simulink model "SpeedControl"  (R2023a)
settings: Solver=FixedStepDiscrete  StartTime=0.0  StopTime=inf  FixedStep=0.02  RelTol=1e-3  EnableMultiTasking=on
undefined symbols (not defined in the file or in its folder): DiscIntNeverNeededParam
libraries: arduinolib x3
settings Model: ExtModeTrigDuration=2  Creator=auw_a  LastModifiedBy=auw_a
settings OptimizationCC: EnhancedBackFolding=on  PassReuseOutputArgsAs=Individual arguments  ZeroExternalMemoryAtStartup=off  ZeroInternalMemoryAtStartup=off  MaxStackSize=64  OptimizeBlockOrder=speed  DifferentSizesBufferReuse=on  OptimizationCustomize=off  EfficientTunableParamExpr=on
settings DebuggingCC: ParameterOverflowMsg=none  ParameterTunabilityLossMsg=error
settings HardwareCC: ProdBitPerPointer=32  ProdBitPerSizeT=32  ProdBitPerPtrDiffT=32  ProdLargestAtomicInteger=Long  ProdLargestAtomicFloat=Double  ProdWordSize=32  ProdHWDeviceType=ARM Compatible->ARM Cortex
settings SFSimCC: MATLABDynamicMemAlloc=off
settings RTWCC: Description=Embedded Coder  SystemTargetFile=ert.tlc  HardwareBoard=ESP32-WROOM(Arduino Compatible)  TLCOptions="-aInlineSetEventsForThisBaseRateFcn=TLC_FALSE -aSuppressMultiTaskScheduler=TLC_FALSE  -aRateBasedStepFcn=0"  TemplateMakefile=ert_default_tmf  Toolchain=ESP32  BuildConfiguration=Faster Runs
settings CodeAppCC: ForceParamTrailComments=on  IgnoreCustomStorageClasses=off  OperatorAnnotations=on  SimulinkDataObjDesc=on  SFDataObjDesc=on  InsertBlockDesc=on
settings ERTTargetCC: SupportContinuousTime=on  SupportVariableSizeSignals=on  ExtModeTransport=3  ExtModeStaticAlloc=on  ExtModeAutomaticAllocSize=off  ExtModeStaticAllocSize=65536  ExtModeMexFile=ext_xcp  ExtModeIntrfLevel=Level2 - Open

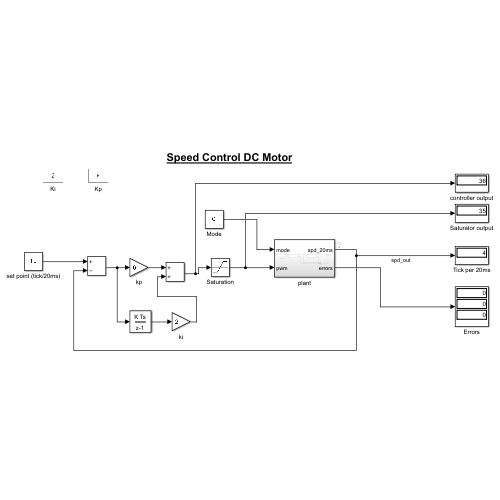
[thumbnail: Simulink's stored preview of the top-level diagram]
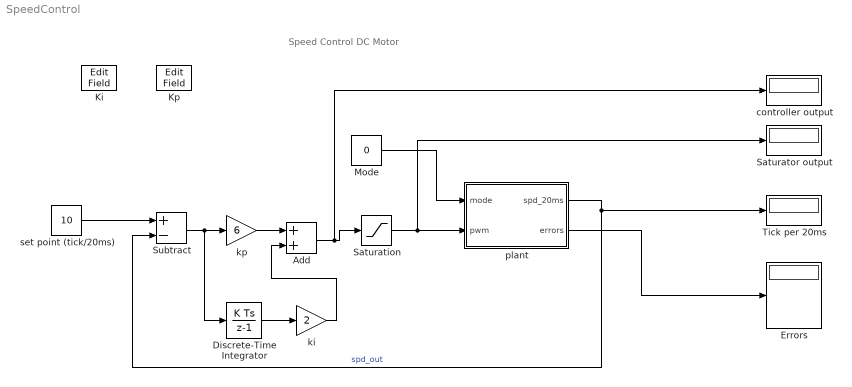
== system SpeedControl ==
  note: Speed Control DC Motor
  Add : Sum
  Discrete-Time Integrator : DiscreteIntegrator  SampleTime=0.02  ICPrevOutput=DiscIntNeverNeededParam  ICPrevScaledInput=DiscIntNeverNeededParam
  Errors : Display
  Ki : EditField  LabelPosition=Hide  ShowInitialText=on  Alignment=Center
  Kp : EditField  LabelPosition=Hide  ShowInitialText=on  Alignment=Center
  Mode : Constant  Value=0
  Saturation : Saturate  UpperLimit=127  LowerLimit=0  OutDataTypeStr=int8
  Saturator output : Display
  Subtract : Sum  Inputs=+-
  Tick per 20ms : Display
  controller output : Display
  ki : Gain  Gain=2
  kp : Gain  Gain=6
  plant : Subsystem
  set point (tick/20ms) : Constant  Value=10  OutDataTypeStr=int8
  wires:
  Mode/1 -> plant/1(mode)
  Saturation/1 -> Saturator output/1, plant/2(pwm)
  plant/1(spd_20ms) -> Subtract/2, Tick per 20ms/1  "spd_out"
  plant/2(errors) -> Errors/1
  set point (tick/20ms)/1 -> Subtract/1
  Subtract/1 -> Discrete-Time Integrator/1, kp/1
  Discrete-Time Integrator/1 -> ki/1
  kp/1 -> Add/1
  Add/1 -> controller output/1, Saturation/1
  ki/1 -> Add/2

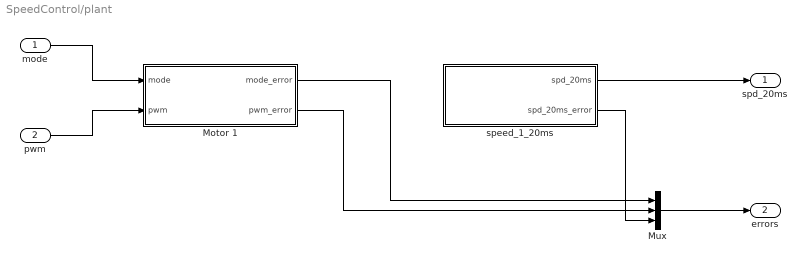
== system SpeedControl/plant ==
  mode : Inport
  pwm : Inport  Port=2
  Motor 1 : Subsystem
  Mux : Mux  Inputs=3
  speed_1_20ms : Subsystem
  spd_20ms : Outport
  errors : Outport  Port=2
  wires:
  Motor 1/2(pwm_error) -> Mux/2
  Motor 1/1(mode_error) -> Mux/1
  speed_1_20ms/2(spd_20ms_error) -> Mux/3
  speed_1_20ms/1(spd_20ms) -> spd_20ms/1
  Mux/1 -> errors/1
  mode/1 -> Motor 1/1(mode)
  pwm/1 -> Motor 1/2(pwm)

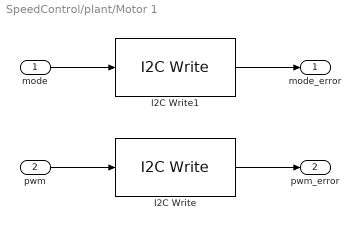
== system SpeedControl/plant/Motor 1 ==
  mode : Inport
  pwm : Inport  Port=2
  I2C Write : arduinolib/I2C Write  I2CModule=0  Mode=Master  SlaveAddress=uint8(hex2dec('24'))  SlaveByteOrder=BigEndian  Direction=Transmitter  RegisterAddressMode=on  RegisterAddress=uint8(hex2dec('20')) + 0  SlaveDataType=uint8  DataLength=1  NoAck=off  RepeatedStart=off  OutputStatus=on  blockPlatform=ARDUINO
  I2C Write1 : arduinolib/I2C Write  I2CModule=0  Mode=Master  SlaveAddress=uint8(hex2dec('24'))  SlaveByteOrder=BigEndian  Direction=Transmitter  RegisterAddressMode=on  RegisterAddress=uint8(hex2dec('60')) + 0  SlaveDataType=uint8  DataLength=1  NoAck=off  RepeatedStart=off  OutputStatus=on  blockPlatform=ARDUINO
  mode_error : Outport
  pwm_error : Outport  Port=2
  wires:
  mode/1 -> I2C Write1/1
  pwm/1 -> I2C Write/1
  I2C Write1/1 -> mode_error/1
  I2C Write/1 -> pwm_error/1

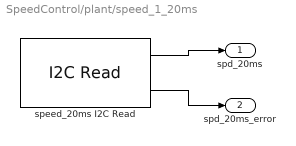
== system SpeedControl/plant/speed_1_20ms ==
  speed_20ms I2C Read : arduinolib/I2C Read  I2CModule=0  Mode=Master  SlaveAddress=uint8(hex2dec('24'))  SlaveByteOrder=BigEndian  Direction=Receiver  RegisterAddressMode=on  RegisterAddress=uint8(hex2dec('40')) + 0  SlaveDataType=int8  DataLength=1  NoAck=off  RepeatedStart=off  OutputStatus=on  blockPlatform=ARDUINO  SampleTime=0.02
  spd_20ms : Outport
  spd_20ms_error : Outport  Port=2
  wires:
  speed_20ms I2C Read/2 -> spd_20ms_error/1
  speed_20ms I2C Read/1 -> spd_20ms/1
